simulink model "Lab_6_Part_three"  (R2015a)
settings: Solver=ode3  StartTime=0.0  StopTime=inf  RelTol=1e-3  SampleTimeConstraint=Specified
libraries: MinSegLibrary_MinSegMega x2, simulink x1
settings Model: SimulationMode=external  ExtModeTrigDuration=2  Creator=009768408  LastModifiedBy=009768408
settings OptimizationCC: OptimizeModelRefInitCode=on  LifeSpan=1
settings DebuggingCC: UnderspecifiedInitializationDetection=Classic  MergeDetectMultiDrivingBlocksExec=none
settings HardwareCC: ProdBitPerInt=16  ProdBitPerPointer=8  ProdIntDivRoundTo=Zero  ProdEndianess=LittleEndian  ProdWordSize=8  ProdHWDeviceType=Atmel->AVR
settings RTWCC: SystemTargetFile=realtime.tlc  GenerateMakefile=off  TemplateMakefile=realtime.tmf  Description=Run on Target Hardware  RTWVerbose=off
settings ERTTargetCC: CombineOutputUpdateFcns=off  ExtModeTransport=3  ExtModeMexFile=ext_serial_win32_comm_rtt  ExtModeMexArgs=0 1 9600  ERTSrcFileBannerTemplate=realtime_code_template.cgt  ERTHdrFileBannerTemplate=realtime_code_template.cgt  ERTDataSrcFileTemplate=realtime_code_template.cgt  ERTDataHdrFileTemplate=realtime_code_template.cgt  ERTCustomFileTemplate=realtime_file_process.tlc

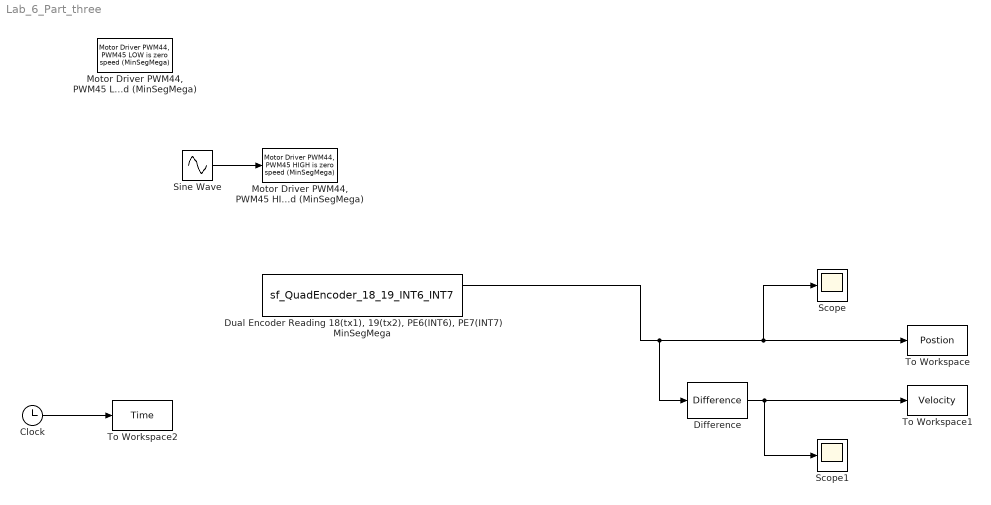
== system Lab_6_Part_three ==
  Clock : Clock
  Difference : simulink/Discrete/Difference  ICPrevInput=0.0  InputProcessing=Inherited  OutMin=[]  OutMax=[]  OutDataType=fixdt(1, 16)  OutScaling=2^-10  DoSatur=off
  "Dual Encoder Reading 18(tx1), 19(tx2), PE6(INT6), PE7(INT7) MinSegMega " : S-Function  InitFcn=try, set_param(gcb,'FunctionName','sf_QuadEncoder_18_19_INT6_INT7'), end  FunctionName=sf_QuadEncoder_18_19_INT6_INT7  Parameters=uint8([0 1]),uint8([18 6]),uint8([19 7])  SFunctionModules=sf_QuadEncoder_18_19_INT6_INT7_wrapper  mask(S-Function Builder){}
      mask init:
      | val = [[.9  0.75 0.75 1 1 .9 .9 1]',[1 1 0.75 0.75 .9 .9 1 .9]'];try , sys = get_param(gcb,'SfunBuilderFcnName');if isempty(sys), sys = get_param(gcb,'FunctionName'); end,catch, sys = get_param(gcb,'FunctionName'); end
      settings: CopyFcn=set_param(gcbh,'LinkStatus','none')  PreSaveFcn=try, set_param(gcb,'FunctionName','sf_QuadEncoder_18_19_INT6_INT7'), end  OpenFcn=sfunctionwizard(gcbh)
      mask Display: plot(val(:,1),val(:,2)),disp(sys), port_label('output',1,'pos1'), port_label('output',2,'pos2')
  "Motor Driver PWM44, PWM45 HIGH is zero speed (MinSegMega)" : MinSegLibrary_MinSegMega/Motor Driver PWM44, PWM45 HIGH is zero speed (MinSegMega)
  "Motor Driver PWM44, PWM45 LOW is zero speed (MinSegMega)" : MinSegLibrary_MinSegMega/Motor Driver PWM44, PWM45 LOW is zero speed (MinSegMega)
  Scope : Scope
  Scope1 : Scope
  Sine Wave : Sin  Amplitude=4.5  Frequency=2  SampleTime=0
  To Workspace : ToWorkspace  VariableName=Postion  SampleTime=-1
  To Workspace1 : ToWorkspace  VariableName=Velocity  SampleTime=-1
  To Workspace2 : ToWorkspace  VariableName=Time  SampleTime=-1
  wires:
  "Dual Encoder Reading 18(tx1), 19(tx2), PE6(INT6), PE7(INT7) MinSegMega "/1 -> Difference/1, Scope/1, To Workspace/1
  Difference/1 -> Scope1/1, To Workspace1/1
  Clock/1 -> To Workspace2/1
  Sine Wave/1 -> "Motor Driver PWM44, PWM45 HIGH is zero speed (MinSegMega)"/1
